simulink library "MotionBaseAdaptersLib"  (R2019b)
settings: Solver=VariableStepAuto  StartTime=0.0  StopTime=10.0  RelTol=1e-3
undefined symbols (not defined in the file): AngularAcceleration, AngularVelocity, ApplyMotion, DiscIntNeverNeededParam, GravitationalAcceleration, LinearAcceleration, LinearVelocity, ManualOrientation, ManualPosition, OrientationDCM, SampleTime, TrackEffectType
libraries: simulink x34, FiltersLib x34, OverridesLib x10, SignalGeneratorsLib x7, LatchesLib x6, TimersLib x5, CoordinateMathOperationsLib x2, MathOperationsLib x2, $bdroot x1
(part 1 of 2)
settings Model: ModifiedComment=azadegaw -- Fri Jun 17 14:06:01 2022 -- Version 1.36  Creator=dward  LastModifiedBy=azadegaw
settings Model: ModifiedHistory=|
  | azadegaw -- Fri Jun 17 14:06:01 2022 -- Version 1.36
  | 
  | azadegaw -- Tue Jun 07 14:53:46 2022 -- Version 1.35
  | added vertical Jolt down.
  | 
  | azadegaw -- Mon Jun 06 18:29:13 2022 -- Version 1.34
  | added absolute to test increase for jolt.
  | multiplied output by input to retain sign,
  | as some jolts are plus and some are minus
  | 
  | staudes -- Thu Apr 21 11:16:42 2022 -- Version 1.33
  | 
  | staudes -- Wed Apr 13 16:31:53 2022 -- Version 1.
  | 
  | staudes -- Thu Apr 07 10:46:09 2022 -- Version 1.31
  | 
  | staudes -- Wed Apr 06 11:32:24 2022 -- Version 1.30
  | Removed Steering Wheel Library
  | 
  | cdyer -- Wed Feb 27 14:51:59 2019 -- Version 1.29
  | - Some modifications to the standard road feel to make it a bit more noticeable
  | - Added logic to lower (and subsequently rampe up) the satuations on accelerations/velocities during collisions
  | - Now set Apply Motion to 0 when Model Data is invalid (mostly handles the extra situation where truksim has stopped the run)
  | 
  | 
  | cdyer -- Wed Feb 20 11:35:48 2019 -- Version 1.28
  | - fixing speed dependent ramp in of motion base effects for raod feel
  | - adding a placeholder for collision gain of motion base outputs
  | 
  | cdyer -- Thu Feb 14 18:34:25 2019 -- Version 1.27
  | -fixed mixup of standard and degraded road feel
  | 
  | cdyer -- Thu Feb 14 12:50:13 2019 -- Version 1.26
  | - Now using the degraded road effect signal to enable the degraded road feel
  | - enabling standard feel by default
  | - road effect may be disabled by setting the profile type to -1.
  | 
  | cdyer -- Wed Jan 16 10:51:13 2019 -- Version 1.25
  | - Adding more complex roughness generation profiles, only enabled by debug properties at this stage
  | 
  | cdyer -- Fri Apr 06 16:05:50 2018 -- Version 1.24
  | -updating default paramaters of steeringwheel adapter for more manageable fualt levels
  | 
  | cdyer -- Thu Feb 15 13:59:35 2018 -- Version 1.23
  | - Adding power steering failure to the effects bus
  | 
  | cdyer -- Mon Jan 22 16:33:43 2018 -- Version 1.22
  | - Upgrading to 2017b
settings DataIOCC: ReturnWorkspaceOutputs=off
settings DebuggingCC: ArithmeticOperatorsInVariantConditions=warning
settings SFSimCC: SimUseLocalCustomCode=off  CustomCodeUndefinedFunction=UseInterfaceOnly
settings RTWCC: RTWUseLocalCustomCode=off
settings CodeAppCC: StateflowObjectComments=on

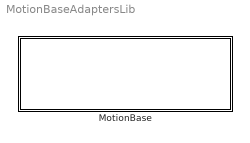
== system MotionBaseAdaptersLib ==
  MotionBase : Subsystem

== system MotionBaseAdaptersLib/MotionBase ==
  MotionBaseAdapter : Subsystem  mask(Motion Base Adapter){}
      mask help: Takes model dynamics data, applies safety limits and outputs motion base control information
  MotionBaseAdaptorInterface : Subsystem

== system MotionBaseAdaptersLib/MotionBase/MotionBaseAdapter ==
  MotionBaseInput : Inport
  Bus to Vector : BusToVector
  MotionBaseProcessing : Subsystem
  SafeMotionBaseOut : Subsystem
  Switch1 : Switch  Criteria=u2 > Threshold
  MotionBaseOutputs : Outport  VectorParamsAs1DForOutWhenUnconnected=off
  StopConditionData : Outport  Port=2  VectorParamsAs1DForOutWhenUnconnected=off
  wires:
  MotionBaseInput/1 -> MotionBaseProcessing/1(MotionBaseInput)
  SafeMotionBaseOut/1(MotionBaseOutputs) -> Switch1/3
  MotionBaseProcessing/1(MotionBaseOutputs) -> Switch1/1
  MotionBaseProcessing/2(AllowMotion) -> Switch1/2
  Switch1/1 -> MotionBaseOutputs/1
  MotionBaseProcessing/3(StopConditionData) -> Bus to Vector/1
  Bus to Vector/1 -> StopConditionData/1

== system MotionBaseAdaptersLib/MotionBase/MotionBaseAdaptorInterface ==
  MotionBaseInput : Inport
  MotionBasePerVehicle : Subsystem
  StopConditionLogging : Subsystem
  MotionBaseOutputs : Outport  VectorParamsAs1DForOutWhenUnconnected=off
  wires:
  MotionBaseInput/1 -> MotionBasePerVehicle/1(MotionBaseInput)
  MotionBasePerVehicle/1(MotionBaseOutputs) -> MotionBaseOutputs/1
  MotionBasePerVehicle/2(StopConditionData) -> StopConditionLogging/1(StopConditionData)

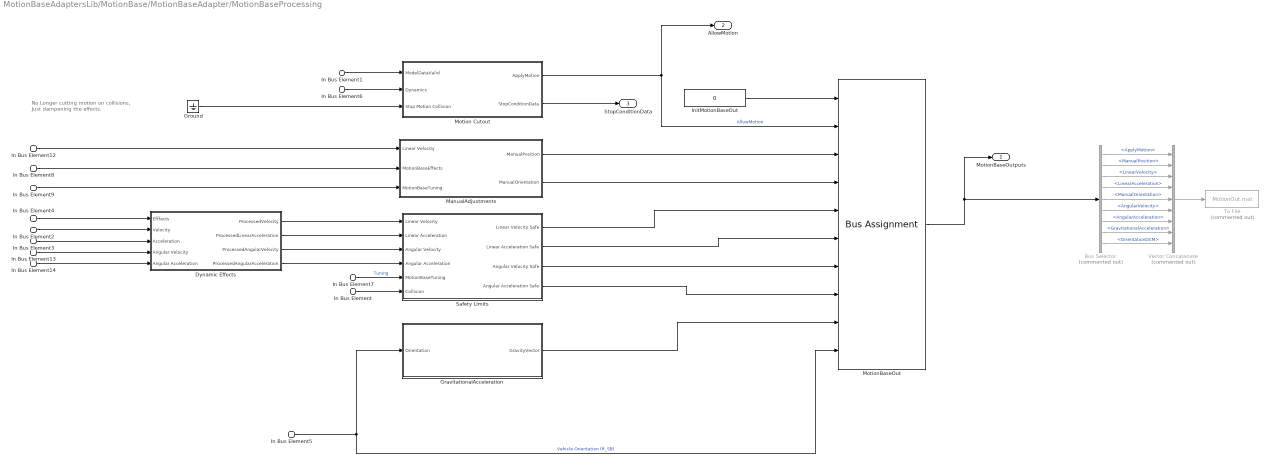
== system MotionBaseAdaptersLib/MotionBase/MotionBaseAdapter/MotionBaseProcessing ==
  note: No Longer cutting motion on collisions,
      | Just dampening the effects.
  In Bus Element : Inport  PortName=MotionBaseInput  Element=Environment.Contact
  In Bus Element6 : Inport  PortName=MotionBaseInput  Element=Dynamics
  In Bus Element12 : Inport  PortName=MotionBaseInput  Element=Dynamics.Velocity
  In Bus Element2 : Inport  PortName=MotionBaseInput  Element=Dynamics.Velocity
  In Bus Element3 : Inport  PortName=MotionBaseInput  Element=Dynamics.Acceleration
  In Bus Element13 : Inport  PortName=MotionBaseInput  Element=Dynamics.AngularVelocity
  In Bus Element14 : Inport  PortName=MotionBaseInput  Element=Dynamics.AngularAcceleration
  In Bus Element5 : Inport  PortName=MotionBaseInput  Element=Dynamics.Transform.OrientationDCM
  In Bus Element4 : Inport  PortName=MotionBaseInput  Element=Effects
  In Bus Element8 : Inport  PortName=MotionBaseInput  Element=Effects.ExternalEffects
  In Bus Element9 : Inport  PortName=MotionBaseInput  Element=Tuning
  In Bus Element7 : Inport  PortName=MotionBaseInput  Element=Tuning
  In Bus Element1 : Inport  PortName=MotionBaseInput  Element=MotionBaseSafetyCutout
  Bus Selector : BusSelector  Commented=on  OutputSignals=ApplyMotion,ManualPosition,LinearVelocity,LinearAcceleration,ManualOrientation,AngularVelocity,AngularAcceleration,GravitationalAcceleration,OrientationDCM
  Dynamic Effects : Subsystem
  GravitationalAcceleration : Subsystem
  Ground : Ground
  InitMotionBaseOut : Constant  Value=0  OutDataTypeStr=Bus: BD_SimIntegration_Out_Vehicle_MotionBaseController
  ManualAdjustments : Subsystem
  Motion Cutout : Subsystem
  MotionBaseOut : BusAssignment  AssignedSignals=ApplyMotion,ManualPosition,ManualOrientation,LinearVelocity,LinearAcceleration,AngularVelocity,AngularAcceleration,GravitationalAcceleration,OrientationDCM
  Safety Limits : Subsystem
  To File : ToFile  Commented=on  Filename=MotionOut.mat  MatrixName=MotionOut
  Vector Concatenate : Concatenate  Commented=on  NumInputs=9
  MotionBaseOutputs : Outport  VectorParamsAs1DForOutWhenUnconnected=off
  AllowMotion : Outport  Port=2  VectorParamsAs1DForOutWhenUnconnected=off
  StopConditionData : Outport  Port=3  VectorParamsAs1DForOutWhenUnconnected=off
  wires:
  In Bus Element1/1 -> Motion Cutout/1(ModelDataValid)
  In Bus Element4/1 -> Dynamic Effects/1(Efffects)
  In Bus Element12/1 -> ManualAdjustments/1(Linear Velocity)
  Dynamic Effects/4(ProcessedAngularAcceleration) -> Safety Limits/4(Angular Acceleration)
  Dynamic Effects/3(ProcessedAngularVelocity) -> Safety Limits/3(Angular Velocity)
  In Bus Element7/1 -> Safety Limits/5(MotionBaseTuning)  "Tuning"
  Dynamic Effects/1(ProcessedVelocity) -> Safety Limits/1(Linear Velocity)
  In Bus Element/1 -> Safety Limits/6(Collision)
  In Bus Element14/1 -> Dynamic Effects/5(Angular Acceleration)
  In Bus Element13/1 -> Dynamic Effects/4(Angular Velocity)
  Dynamic Effects/2(ProcessedLinearAcceleration) -> Safety Limits/2(Linear Acceleration)
  Ground/1 -> Motion Cutout/3(Stop Motion Collision)
  In Bus Element8/1 -> ManualAdjustments/2(MotionBaseEffects)
  In Bus Element9/1 -> ManualAdjustments/3(MotionBaseTuning)
  InitMotionBaseOut/1 -> MotionBaseOut/1
  Motion Cutout/1(ApplyMotion) -> AllowMotion/1, MotionBaseOut/2  "AllowMotion"
  In Bus Element3/1 -> Dynamic Effects/3(Acceleration)
  MotionBaseOut/1 -> Bus Selector/1, MotionBaseOutputs/1
  In Bus Element5/1 -> GravitationalAcceleration/1(Orientation), MotionBaseOut/10  "Vehicle Orientation (R_SB)"
  In Bus Element2/1 -> Dynamic Effects/2(Velocity)
  Safety Limits/1(Linear Velocity Safe) -> MotionBaseOut/5
  Safety Limits/2(Linear Acceleration Safe) -> MotionBaseOut/6
  Safety Limits/3(Angular Velocity Safe) -> MotionBaseOut/7
  Safety Limits/4(Angular Acceleration Safe) -> MotionBaseOut/8
  Bus Selector/5 -> Vector Concatenate/5  "<ManualOrientation>"
  Bus Selector/2 -> Vector Concatenate/2  "<ManualPosition>"
  Bus Selector/4 -> Vector Concatenate/4  "<LinearAcceleration>"
  Bus Selector/6 -> Vector Concatenate/6  "<AngularVelocity>"
  Bus Selector/7 -> Vector Concatenate/7  "<AngularAcceleration>"
  Bus Selector/9 -> Vector Concatenate/9  "<OrientationDCM>"
  Vector Concatenate/1 -> To File/1
  Bus Selector/3 -> Vector Concatenate/3  "<LinearVelocity>"
  Bus Selector/1 -> Vector Concatenate/1  "<ApplyMotion>"
  Bus Selector/8 -> Vector Concatenate/8  "<GravitationalAcceleration>"
  In Bus Element6/1 -> Motion Cutout/2(Dynamics)
  Motion Cutout/2(StopConditionData) -> StopConditionData/1
  GravitationalAcceleration/1(GravityVector) -> MotionBaseOut/9
  ManualAdjustments/1(ManualPosition) -> MotionBaseOut/3
  ManualAdjustments/2(ManualOrientation) -> MotionBaseOut/4

== system MotionBaseAdaptersLib/MotionBase/MotionBaseAdapter/SafeMotionBaseOut ==
  InitMotionBaseOut1 : Constant  Value=0  OutDataTypeStr=Bus: BD_SimIntegration_Out_Vehicle_MotionBaseController
  SafeGravitationalAcceleration : Constant  Value=[0 0 -9.81]
  SafeMotionBaseOut : BusAssignment  AssignedSignals=GravitationalAcceleration,OrientationDCM
  SafeRotationMatrix : Constant  Value=eye(3)
  MotionBaseOutputs : Outport  VectorParamsAs1DForOutWhenUnconnected=off
  wires:
  SafeRotationMatrix/1 -> SafeMotionBaseOut/3
  SafeMotionBaseOut/1 -> MotionBaseOutputs/1  "SafeMotionBaseOut"
  InitMotionBaseOut1/1 -> SafeMotionBaseOut/1
  SafeGravitationalAcceleration/1 -> SafeMotionBaseOut/2

== system MotionBaseAdaptersLib/MotionBase/MotionBaseAdaptorInterface/MotionBasePerVehicle ==
  MotionBaseInput : Inport  Partition=on  PartitionDimension=1  PartitionWidth=1  PartitionOffset=0
  For Each : ForEach  DisableCoverage=on
  MotionBaseAdapter : $bdroot/MotionBase/MotionBaseAdapter
  MotionBaseOutputs : Outport  ConcatenationDimension=1  VectorParamsAs1DForOutWhenUnconnected=off
  StopConditionData : Outport  Port=2  ConcatenationDimension=1  VectorParamsAs1DForOutWhenUnconnected=off
  wires:
  MotionBaseInput/1 -> MotionBaseAdapter/1
  MotionBaseAdapter/2 -> StopConditionData/1
  MotionBaseAdapter/1 -> MotionBaseOutputs/1

== system MotionBaseAdaptersLib/MotionBase/MotionBaseAdaptorInterface/StopConditionLogging ==
  StopConditionData : Inport
  Data Type Conversion : DataTypeConversion
  Demux : Demux  Outputs=5
  Log On Stop Motion : Subsystem  TreatAsAtomicUnit=on
  Vector Concatenate : Concatenate  NumInputs=4
  wires:
  Demux/5 -> Vector Concatenate/4
  Demux/1 -> Log On Stop Motion/Enable
  Demux/4 -> Vector Concatenate/3
  Data Type Conversion/1 -> Log On Stop Motion/1(In1)
  Vector Concatenate/1 -> Data Type Conversion/1
  Demux/2 -> Vector Concatenate/1
  Demux/3 -> Vector Concatenate/2
  StopConditionData/1 -> Demux/1

== system MotionBaseAdaptersLib/MotionBase/MotionBaseAdapter/MotionBaseProcessing/Dynamic Effects ==
  Efffects : Inport
  Velocity : Inport  Port=2
  Acceleration : Inport  Port=3
  Angular Velocity : Inport  Port=4
  Angular Acceleration : Inport  Port=5
  Acceleration Jolts : Subsystem
  ProcessedVelocity : Outport
  ProcessedLinearAcceleration : Outport  Port=2
  ProcessedAngularVelocity : Outport  Port=3
  ProcessedAngularAcceleration : Outport  Port=4
  wires:
  Angular Acceleration/1 -> ProcessedAngularAcceleration/1
  Angular Velocity/1 -> ProcessedAngularVelocity/1
  Velocity/1 -> ProcessedVelocity/1
  Efffects/1 -> Acceleration Jolts/1(Effects)
  Acceleration Jolts/1(AccelerationOut) -> ProcessedLinearAcceleration/1
  Acceleration/1 -> Acceleration Jolts/2(AccelerationIn)

== system MotionBaseAdaptersLib/MotionBase/MotionBaseAdapter/MotionBaseProcessing/GravitationalAcceleration ==
  Orientation : Inport
  DCM Invert : CoordinateMathOperationsLib/DCM Invert
      settings: SourceProductName=Coordinate Systems
  DCM Multiply : CoordinateMathOperationsLib/DCM Multiply
      settings: SourceProductName=Coordinate Systems
  GravitationalAcceleration : Constant  Value=[0 0 -9.81]
  GravityVector : Outport  VectorParamsAs1DForOutWhenUnconnected=off
  wires:
  GravitationalAcceleration/1 -> DCM Multiply/2  "Accleration do to Gravity (V_S)"
  DCM Invert/1 -> DCM Multiply/1  "Vehicle Orientation (R_BS"
  DCM Multiply/1 -> GravityVector/1
  Orientation/1 -> DCM Invert/1

== system MotionBaseAdaptersLib/MotionBase/MotionBaseAdapter/MotionBaseProcessing/ManualAdjustments ==
  Linear Velocity : Inport
  MotionBaseEffects : Inport  Port=2
  MotionBaseTuning : Inport  Port=3
  ManualOrientationAdjustment : Constant  Value=[0 0 0]
  ManualPositionAdjustment : Subsystem
  ManualPositionAdjustment1 : Subsystem  Commented=on
  ManualPosition : Outport  VectorParamsAs1DForOutWhenUnconnected=off
  ManualOrientation : Outport  Port=2  VectorParamsAs1DForOutWhenUnconnected=off
  wires:
  MotionBaseEffects/1 -> ManualPositionAdjustment/2(MotionBaseEffects)
  Linear Velocity/1 -> ManualPositionAdjustment/1(Linear Velocity)
  MotionBaseTuning/1 -> ManualPositionAdjustment/3(MotionBaseTuning)
  ManualOrientationAdjustment/1 -> ManualOrientation/1  "ManualOrientation"
  ManualPositionAdjustment/1(ManualPosition) -> ManualPosition/1  "ManualPosition"

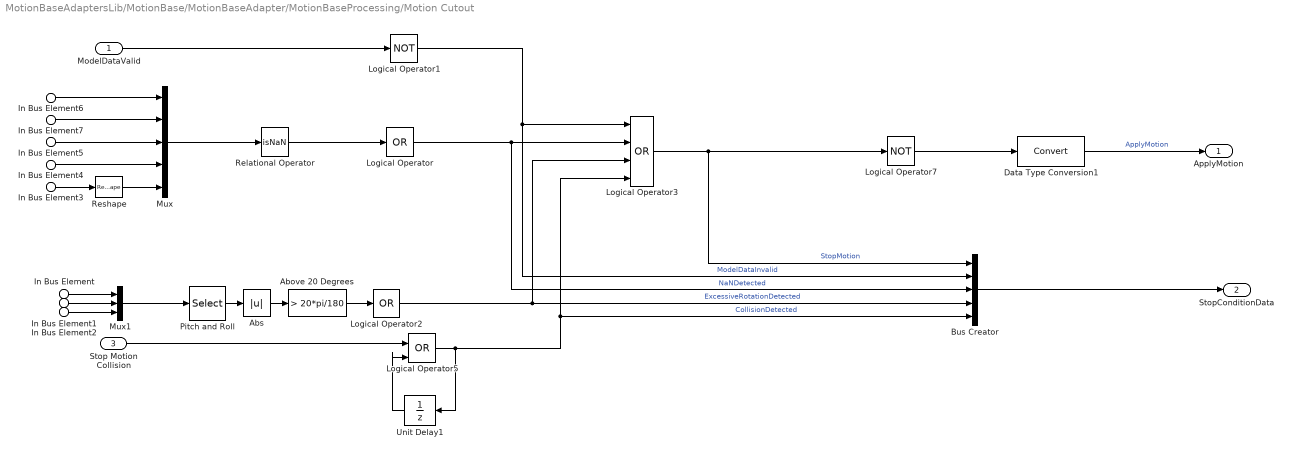
== system MotionBaseAdaptersLib/MotionBase/MotionBaseAdapter/MotionBaseProcessing/Motion Cutout ==
  ModelDataValid : Inport
  In Bus Element : Inport  Port=2  PortName=Dynamics  Element=Transform.H
  In Bus Element1 : Inport  Port=2  PortName=Dynamics  Element=Transform.P
  In Bus Element2 : Inport  Port=2  PortName=Dynamics  Element=Transform.R
  In Bus Element3 : Inport  Port=2  PortName=Dynamics  Element=Transform.OrientationDCM
  In Bus Element4 : Inport  Port=2  PortName=Dynamics  Element=AngularAcceleration
  In Bus Element5 : Inport  Port=2  PortName=Dynamics  Element=AngularVelocity
  In Bus Element6 : Inport  Port=2  PortName=Dynamics  Element=Velocity
  In Bus Element7 : Inport  Port=2  PortName=Dynamics  Element=Acceleration
  Stop Motion Collision : Inport  Port=3
  Above 20 Degrees : simulink/Logic and Bit Operations/Compare To Constant  relop=>  const=20*pi/180  OutDataTypeStr=boolean
  Abs : Abs
  Bus Creator : BusCreator  Inputs=5
  Data Type Conversion1 : DataTypeConversion
  Logical Operator : Logic  Operator=OR  Inputs=1  IconShape=distinctive  AllPortsSameDT=off  OutDataTypeStr=boolean
  Logical Operator1 : Logic  Operator=NOT  IconShape=distinctive  AllPortsSameDT=off  OutDataTypeStr=boolean
  Logical Operator2 : Logic  Operator=OR  Inputs=1  IconShape=distinctive  AllPortsSameDT=off  OutDataTypeStr=boolean
  Logical Operator3 : Logic  Operator=OR  Inputs=4  IconShape=distinctive  AllPortsSameDT=off  OutDataTypeStr=boolean
  Logical Operator5 : Logic  Operator=OR  IconShape=distinctive  AllPortsSameDT=off  OutDataTypeStr=boolean
  Logical Operator7 : Logic  Operator=NOT  IconShape=distinctive  AllPortsSameDT=off  OutDataTypeStr=boolean
  Mux : Mux  Inputs=[3 3 3 3 9]
  Mux1 : Mux  Inputs=3
  Pitch and Roll : Selector  InputPortWidth=3  IndexOptions=Index vector (dialog)  Indices=[2 3]  OutputSizes=1
  Relational Operator : RelationalOperator  Operator=isNaN  OutDataTypeStr=boolean  RndMeth=Nearest
  Reshape : Reshape
  Unit Delay1 : UnitDelay  SampleTime=-1  HasFrameUpgradeWarning=on
  ApplyMotion : Outport  VectorParamsAs1DForOutWhenUnconnected=off
  StopConditionData : Outport  Port=2  VectorParamsAs1DForOutWhenUnconnected=off
  wires:
  Logical Operator1/1 -> Logical Operator3/1, Bus Creator/2  "ModelDataInvalid"
  ModelDataValid/1 -> Logical Operator1/1
  Stop Motion Collision/1 -> Logical Operator5/1
  Logical Operator3/1 -> Bus Creator/1, Logical Operator7/1  "StopMotion"
  Mux/1 -> Relational Operator/1
  Relational Operator/1 -> Logical Operator/1
  Logical Operator/1 -> Bus Creator/3, Logical Operator3/2  "NaNDetected"
  In Bus Element6/1 -> Mux/1
  In Bus Element5/1 -> Mux/3
  In Bus Element3/1 -> Reshape/1
  In Bus Element4/1 -> Mux/4
  In Bus Element7/1 -> Mux/2
  Abs/1 -> Above 20 Degrees/1
  Above 20 Degrees/1 -> Logical Operator2/1
  Logical Operator2/1 -> Bus Creator/4, Logical Operator3/3  "ExcessiveRotationDetected"
  Pitch and Roll/1 -> Abs/1
  Logical Operator5/1 -> Unit Delay1/1, Bus Creator/5, Logical Operator3/4  "CollisionDetected"
  Unit Delay1/1 -> Logical Operator5/2
  Logical Operator7/1 -> Data Type Conversion1/1
  Data Type Conversion1/1 -> ApplyMotion/1  "ApplyMotion"
  In Bus Element2/1 -> Mux1/3
  In Bus Element1/1 -> Mux1/2
  In Bus Element/1 -> Mux1/1
  Mux1/1 -> Pitch and Roll/1
  Reshape/1 -> Mux/5
  Bus Creator/1 -> StopConditionData/1

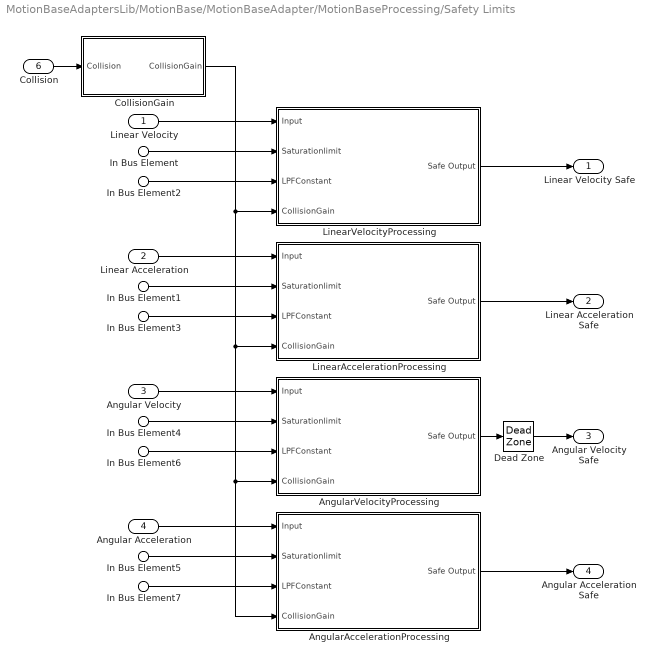
== system MotionBaseAdaptersLib/MotionBase/MotionBaseAdapter/MotionBaseProcessing/Safety Limits ==
  Linear Velocity : Inport
  Linear Acceleration : Inport  Port=2
  Angular Velocity : Inport  Port=3
  Angular Acceleration : Inport  Port=4
  In Bus Element : Inport  Port=5  PortName=MotionBaseTuning  Element=LinearVelocitySaturation
  In Bus Element1 : Inport  Port=5  PortName=MotionBaseTuning  Element=LinearAccelerationSaturation
  In Bus Element2 : Inport  Port=5  PortName=MotionBaseTuning  Element=LinearVelocityLPFConstant
  In Bus Element3 : Inport  Port=5  PortName=MotionBaseTuning  Element=LinearAccelerationLPFConstant
  In Bus Element4 : Inport  Port=5  PortName=MotionBaseTuning  Element=AngularVelocitySaturation
  In Bus Element5 : Inport  Port=5  PortName=MotionBaseTuning  Element=AngularAccelerationSaturation
  In Bus Element6 : Inport  Port=5  PortName=MotionBaseTuning  Element=AngularVelocityLPFConstant
  In Bus Element7 : Inport  Port=5  PortName=MotionBaseTuning  Element=AngularAccelerationLPFConstant
  Collision : Inport  Port=6
  AngularAccelerationProcessing : Subsystem
  AngularVelocityProcessing : Subsystem
  CollisionGain : Subsystem
  Dead Zone : DeadZone  LowerValue=-1e-05  UpperValue=1e-05  SaturateOnIntegerOverflow=on
  LinearAccelerationProcessing : Subsystem
  LinearVelocityProcessing : Subsystem
  Linear Velocity Safe : Outport  VectorParamsAs1DForOutWhenUnconnected=off
  Linear Acceleration Safe : Outport  Port=2  VectorParamsAs1DForOutWhenUnconnected=off
  Angular Velocity Safe : Outport  Port=3  VectorParamsAs1DForOutWhenUnconnected=off
  Angular Acceleration Safe : Outport  Port=4  VectorParamsAs1DForOutWhenUnconnected=off
  wires:
  Collision/1 -> CollisionGain/1(Collision)
  CollisionGain/1(CollisionGain) -> LinearAccelerationProcessing/4(CollisionGain), AngularAccelerationProcessing/4(CollisionGain), AngularVelocityProcessing/4(CollisionGain), LinearVelocityProcessing/4(CollisionGain)
  In Bus Element7/1 -> AngularAccelerationProcessing/3(LPFConstant)
  In Bus Element6/1 -> AngularVelocityProcessing/3(LPFConstant)
  In Bus Element5/1 -> AngularAccelerationProcessing/2(Saturationlimit)
  In Bus Element4/1 -> AngularVelocityProcessing/2(Saturationlimit)
  In Bus Element1/1 -> LinearAccelerationProcessing/2(Saturationlimit)
  In Bus Element/1 -> LinearVelocityProcessing/2(Saturationlimit)
  Linear Velocity/1 -> LinearVelocityProcessing/1(Input)
  In Bus Element2/1 -> LinearVelocityProcessing/3(LPFConstant)
  LinearVelocityProcessing/1(Safe Output) -> Linear Velocity Safe/1
  In Bus Element3/1 -> LinearAccelerationProcessing/3(LPFConstant)
  Linear Acceleration/1 -> LinearAccelerationProcessing/1(Input)
  LinearAccelerationProcessing/1(Safe Output) -> Linear Acceleration Safe/1
  Angular Velocity/1 -> AngularVelocityProcessing/1(Input)
  AngularVelocityProcessing/1(Safe Output) -> Dead Zone/1
  Dead Zone/1 -> Angular Velocity Safe/1
  AngularAccelerationProcessing/1(Safe Output) -> Angular Acceleration Safe/1
  Angular Acceleration/1 -> AngularAccelerationProcessing/1(Input)

== system MotionBaseAdaptersLib/MotionBase/MotionBaseAdaptorInterface/StopConditionLogging/Log On Stop Motion ==
  In1 : Inport
  Enable : EnablePort
  To File : ToFile  Filename=MotionStop.mat  MatrixName=MotionStop
  wires:
  In1/1 -> To File/1

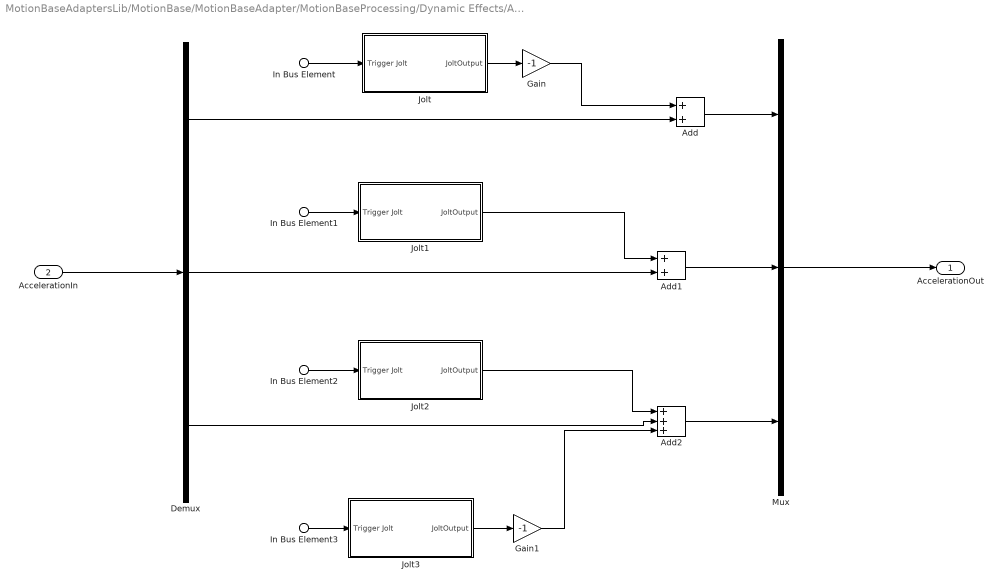
== system MotionBaseAdaptersLib/MotionBase/MotionBaseAdapter/MotionBaseProcessing/Dynamic Effects/Acceleration Jolts ==
  In Bus Element : Inport  PortName=Effects  Element=LongitudinalJolt
  In Bus Element1 : Inport  PortName=Effects  Element=LateralJolt
  In Bus Element2 : Inport  PortName=Effects  Element=VerticalJolt
  In Bus Element3 : Inport  PortName=Effects  Element=VerticalJoltDown
  AccelerationIn : Inport  Port=2
  Add : Sum
  Add1 : Sum
  Add2 : Sum  Inputs=+++
  Demux : Demux  Outputs=3
  Gain : Gain  Gain=-1
  Gain1 : Gain  Gain=-1
  Jolt : Subsystem  mask{Duration=0.5, JoltProfile=[0, 1.5, 2, 1.8, 1.5, 0], JoltBreakPoints=[0, 0.1, 0.2, 0.3, 0.4, 0.5]}
      mask prompts: Duration "Duration of Jolt"; JoltProfile "Jolt Profile Curve"; JoltBreakPoints "Jolt Breakpoints"
      mask help:
      | Creates a disturbance with a specified profile upon a rising edge of the input.
      |
      | Duration must be equal to the end time specified in the Jolt Breakpoints in order for the signal to work correctly
  Jolt1 : Subsystem  mask{Duration=0.5, JoltProfile=[0, 1.5, 2, 1.8, 1.5, 0], JoltBreakPoints=[0, 0.1, 0.2, 0.3, 0.4, 0.5]}
      mask prompts: Duration "Duration of Jolt"; JoltProfile "Jolt Profile Curve"; JoltBreakPoints "Jolt Breakpoints"
      mask help:
      | Creates a disturbance with a specified profile upon a rising edge of the input.
      |
      | Duration must be equal to the end time specified in the Jolt Breakpoints in order for the signal to work correctly
  Jolt2 : Subsystem  mask{Duration=0.5, JoltProfile=[0, 1.5, 2, 1.8, 1.5, 0], JoltBreakPoints=[0, 0.1, 0.2, 0.3, 0.4, 0.5]}
      mask prompts: Duration "Duration of Jolt"; JoltProfile "Jolt Profile Curve"; JoltBreakPoints "Jolt Breakpoints"
      mask help:
      | Creates a disturbance with a specified profile upon a rising edge of the input.
      |
      | Duration must be equal to the end time specified in the Jolt Breakpoints in order for the signal to work correctly
  Jolt3 : Subsystem  mask{Duration=0.5, JoltProfile=[0, 1.5, 2, 1.8, 1.5, 0], JoltBreakPoints=[0, 0.1, 0.2, 0.3, 0.4, 0.5]}
      mask prompts: Duration "Duration of Jolt"; JoltProfile "Jolt Profile Curve"; JoltBreakPoints "Jolt Breakpoints"
      mask help:
      | Creates a disturbance with a specified profile upon a rising edge of the input.
      |
      | Duration must be equal to the end time specified in the Jolt Breakpoints in order for the signal to work correctly
  Mux : Mux  Inputs=3
  AccelerationOut : Outport
  wires:
  Gain1/1 -> Add2/3
  Jolt3/1(JoltOutput) -> Gain1/1
  In Bus Element3/1 -> Jolt3/1(Trigger Jolt)
  Jolt2/1(JoltOutput) -> Add2/1
  Jolt1/1(JoltOutput) -> Add1/1
  Gain/1 -> Add/1
  Jolt/1(JoltOutput) -> Gain/1
  In Bus Element2/1 -> Jolt2/1(Trigger Jolt)
  In Bus Element1/1 -> Jolt1/1(Trigger Jolt)
  In Bus Element/1 -> Jolt/1(Trigger Jolt)
  Mux/1 -> AccelerationOut/1
  AccelerationIn/1 -> Demux/1
  Add2/1 -> Mux/3
  Add/1 -> Mux/1
  Add1/1 -> Mux/2
  Demux/1 -> Add/2
  Demux/2 -> Add1/2
  Demux/3 -> Add2/2

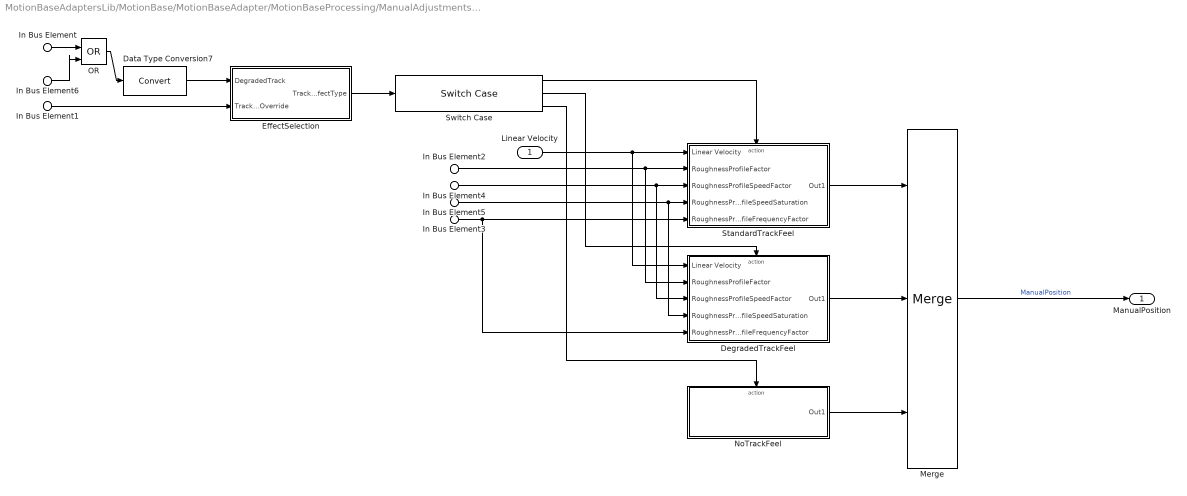
== system MotionBaseAdaptersLib/MotionBase/MotionBaseAdapter/MotionBaseProcessing/ManualAdjustments/ManualPositionAdjustment ==
  Linear Velocity : Inport
  In Bus Element6 : Inport  Port=2  PortName=MotionBaseEffects  Element=DegradedTrack
  In Bus Element : Inport  Port=2  PortName=MotionBaseEffects  Element=OnRoughTrack
  In Bus Element2 : Inport  Port=3  PortName=MotionBaseTuning  Element=RoughnessProfileFactor
  In Bus Element1 : Inport  Port=3  PortName=MotionBaseTuning  Element=RoughnessProfileType
  In Bus Element3 : Inport  Port=3  PortName=MotionBaseTuning  Element=RoughnessProfileFrequencyFactor
  In Bus Element4 : Inport  Port=3  PortName=MotionBaseTuning  Element=RoughnessProfileSpeedFactor
  In Bus Element5 : Inport  Port=3  PortName=MotionBaseTuning  Element=RoughnessProfileSpeedSaturation
  Data Type Conversion7 : DataTypeConversion
  DegradedTrackFeel : Subsystem  TreatAsAtomicUnit=on
  EffectSelection : Subsystem
  Merge : Merge  Inputs=3
  NoTrackFeel : Subsystem  TreatAsAtomicUnit=on
  OR : Logic  Operator=OR  IconShape=distinctive  AllPortsSameDT=off  OutDataTypeStr=boolean
  StandardTrackFeel : Subsystem  TreatAsAtomicUnit=on
  Switch Case : SwitchCase  CaseConditions={TrackEffectType.StandardTrack, TrackEffectType.DegradedTrack, TrackEffectType.NoTrackEffect}  ShowDefaultCase=off
  ManualPosition : Outport  VectorParamsAs1DForOutWhenUnconnected=off
  wires:
  Data Type Conversion7/1 -> EffectSelection/1(DegradedTrack)
  OR/1 -> Data Type Conversion7/1
  In Bus Element/1 -> OR/1
  EffectSelection/1(TrackEffectType) -> Switch Case/1
  In Bus Element6/1 -> OR/2
  In Bus Element1/1 -> EffectSelection/2(TrackEffectOverride)
  Switch Case/2 -> DegradedTrackFeel/Action
  In Bus Element3/1 -> StandardTrackFeel/5(RoughnessProfileFrequencyFactor), DegradedTrackFeel/5(RoughnessProfileFrequencyFactor)
  Linear Velocity/1 -> StandardTrackFeel/1(Linear Velocity), DegradedTrackFeel/1(Linear Velocity)
  DegradedTrackFeel/1(Out1) -> Merge/2
  In Bus Element5/1 -> StandardTrackFeel/4(RoughnessProfileSpeedSaturation), DegradedTrackFeel/4(RoughnessProfileSpeedSaturation)
  In Bus Element4/1 -> StandardTrackFeel/3(RoughnessProfileSpeedFactor), DegradedTrackFeel/3(RoughnessProfileSpeedFactor)
  StandardTrackFeel/1(Out1) -> Merge/1
  In Bus Element2/1 -> StandardTrackFeel/2(RoughnessProfileFactor), DegradedTrackFeel/2(RoughnessProfileFactor)
  NoTrackFeel/1(Out1) -> Merge/3
  Switch Case/3 -> NoTrackFeel/Action
  Switch Case/1 -> StandardTrackFeel/Action
  Merge/1 -> ManualPosition/1  "ManualPosition"

== system MotionBaseAdaptersLib/MotionBase/MotionBaseAdapter/MotionBaseProcessing/ManualAdjustments/ManualPositionAdjustment1 ==
  Linear Velocity : Inport
  In Bus Element2 : Inport  Port=2  PortName=MotionBaseTuning  Element=RoughnessProfileFactor
  In Bus Element1 : Inport  Port=2  PortName=MotionBaseTuning  Element=RoughnessProfileType
  In Bus Element3 : Inport  Port=2  PortName=MotionBaseTuning  Element=RoughnessProfileFrequencyFactor
  In Bus Element4 : Inport  Port=2  PortName=MotionBaseTuning  Element=RoughnessProfileSpeedFactor
  In Bus Element5 : Inport  Port=2  PortName=MotionBaseTuning  Element=RoughnessProfileSpeedSaturation
  If : If  IfExpression=u1 == 1  ElseIfExpressions=u1 == 2,u1 == 3,u1 == 4
  If Action Subsystem : Subsystem  TreatAsAtomicUnit=on
  If Action Subsystem1 : Subsystem  TreatAsAtomicUnit=on
  If Action Subsystem2 : Subsystem  TreatAsAtomicUnit=on
  If Action Subsystem3 : Subsystem  Commented=on  TreatAsAtomicUnit=on
  If Action Subsystem4 : Subsystem  Commented=on  TreatAsAtomicUnit=on
  If Action Subsystem5 : Subsystem  TreatAsAtomicUnit=on
  If Action Subsystem6 : Subsystem  TreatAsAtomicUnit=on
  Merge : Merge  Inputs=5
  ManualPosition : Outport  VectorParamsAs1DForOutWhenUnconnected=off
  wires:
  Merge/1 -> ManualPosition/1  "ManualPosition"
  In Bus Element1/1 -> If/1
  If/1 -> If Action Subsystem/Action
  If/2 -> If Action Subsystem1/Action
  If/5 -> If Action Subsystem2/Action
  If Action Subsystem/1(Out1) -> Merge/1
  If Action Subsystem1/1(Out1) -> Merge/2
  If Action Subsystem2/1(Out1) -> Merge/5
  In Bus Element2/1 -> If Action Subsystem6/2(RoughnessProfileFactor), If Action Subsystem5/2(RoughnessProfileFactor), If Action Subsystem1/2(RoughnessProfileFactor), If Action Subsystem/2(RoughnessProfileFactor)
  If/3 -> If Action Subsystem5/Action
  If Action Subsystem5/1(Out1) -> Merge/3
  In Bus Element4/1 -> If Action Subsystem6/3(RoughnessProfileSpeedFactor), If Action Subsystem5/3(RoughnessProfileSpeedFactor), If Action Subsystem1/3(RoughnessProfileSpeedFactor), If Action Subsystem/3(RoughnessProfileSpeedFactor)
  In Bus Element5/1 -> If Action Subsystem6/4(RoughnessProfileSpeedSaturation), If Action Subsystem5/4(RoughnessProfileSpeedSaturation), If Action Subsystem1/4(RoughnessProfileSpeedSaturation), If Action Subsystem/4(RoughnessProfileSpeedSaturation)
  If/4 -> If Action Subsystem6/Action
  If Action Subsystem6/1(Out1) -> Merge/4
  Linear Velocity/1 -> If Action Subsystem5/1(Linear Velocity), If Action Subsystem6/1(Linear Velocity), If Action Subsystem1/1(Linear Velocity), If Action Subsystem/1(Linear Velocity)
  In Bus Element3/1 -> If Action Subsystem/5(RoughnessProfileFrequencyFactor), If Action Subsystem1/5(RoughnessProfileFrequencyFactor), If Action Subsystem5/5(RoughnessProfileFrequencyFactor), If Action Subsystem6/5(RoughnessProfileFrequencyFactor)

== system MotionBaseAdaptersLib/MotionBase/MotionBaseAdapter/MotionBaseProcessing/Safety Limits/AngularAccelerationProcessing ==
  Input : Inport
  Saturationlimit : Inport  Port=2
  LPFConstant : Inport  Port=3
  CollisionGain : Inport  Port=4
  1-D Lookup Table : Lookup_n-D  NumberOfTableDimensions=1  BreakpointsForDimension1=[.1 1]  Table=[.5 1]  ExtrapMethod=Clip  UseLastTableValue=on  InternalRulePriority=Speed  RndMeth=Simplest  InputSameDT=on
  First Order Low Pass Filter : FiltersLib/First Order Low Pass Filter  FilterSpecificationSource=external  FilterSpecificationType=Specify Cutoff Frequency  FilterSpecificationValue=0.01  SampleTime=-1
      settings: SourceProductName=Filters
  Gain : Gain  Gain=-1
  LPFConstantTuning : OverridesLib/Tuning Factor  DefaultValue=4.5  Criteria=u2 > Threshold  Threshold=0
      settings: SourceProductName=Sydac Utilities
  Product : Product
  Saturation Dynamic : simulink/Discontinuities/Saturation Dynamic  OutMin=[]  OutMax=[]  OutDataTypeStr=Inherit: Same as second input  OutDataType=fixdt(1, 16)  OutScaling=2^-10  DoSatur=off
  SaturationTuning : OverridesLib/Tuning Factor  DefaultValue=2  Criteria=u2 > Threshold  Threshold=0
      settings: SourceProductName=Sydac Utilities
  Safe Output : Outport  VectorParamsAs1DForOutWhenUnconnected=off
  wires:
  1-D Lookup Table/1 -> Product/1
  SaturationTuning/1 -> Product/2
  CollisionGain/1 -> 1-D Lookup Table/1
  LPFConstantTuning/1 -> First Order Low Pass Filter/2
  Saturation Dynamic/1 -> Safe Output/1
  First Order Low Pass Filter/1 -> Saturation Dynamic/2
  Saturationlimit/1 -> SaturationTuning/1
  LPFConstant/1 -> LPFConstantTuning/1
  Input/1 -> First Order Low Pass Filter/1
  Product/1 -> Gain/1, Saturation Dynamic/1
  Gain/1 -> Saturation Dynamic/3

== system MotionBaseAdaptersLib/MotionBase/MotionBaseAdapter/MotionBaseProcessing/Safety Limits/AngularVelocityProcessing ==
  Input : Inport
  Saturationlimit : Inport  Port=2
  LPFConstant : Inport  Port=3
  CollisionGain : Inport  Port=4
  1-D Lookup Table : Lookup_n-D  NumberOfTableDimensions=1  BreakpointsForDimension1=[.1 1]  Table=[.4 1]  ExtrapMethod=Clip  UseLastTableValue=on  InternalRulePriority=Speed  RndMeth=Simplest  InputSameDT=on
  First Order Low Pass Filter : FiltersLib/First Order Low Pass Filter  FilterSpecificationSource=external  FilterSpecificationType=Specify Cutoff Frequency  FilterSpecificationValue=0.01  SampleTime=-1
      settings: SourceProductName=Filters
  Gain : Gain  Gain=-1
  LPFConstantTuning : OverridesLib/Tuning Factor  DefaultValue=10  Criteria=u2 > Threshold  Threshold=0
      settings: SourceProductName=Sydac Utilities
  Product : Product
  Saturation Dynamic : simulink/Discontinuities/Saturation Dynamic  OutMin=[]  OutMax=[]  OutDataTypeStr=Inherit: Same as second input  OutDataType=fixdt(1, 16)  OutScaling=2^-10  DoSatur=off
  SaturationTuning : OverridesLib/Tuning Factor  DefaultValue=2  Criteria=u2 > Threshold  Threshold=0
      settings: SourceProductName=Sydac Utilities
  Safe Output : Outport  VectorParamsAs1DForOutWhenUnconnected=off
  wires:
  1-D Lookup Table/1 -> Product/1
  CollisionGain/1 -> 1-D Lookup Table/1
  SaturationTuning/1 -> Product/2
  LPFConstantTuning/1 -> First Order Low Pass Filter/2
  Saturation Dynamic/1 -> Safe Output/1
  First Order Low Pass Filter/1 -> Saturation Dynamic/2
  Saturationlimit/1 -> SaturationTuning/1
  LPFConstant/1 -> LPFConstantTuning/1
  Input/1 -> First Order Low Pass Filter/1
  Product/1 -> Gain/1, Saturation Dynamic/1
  Gain/1 -> Saturation Dynamic/3

== system MotionBaseAdaptersLib/MotionBase/MotionBaseAdapter/MotionBaseProcessing/Safety Limits/CollisionGain ==
  note: May be able to try and dampen the motion base repsonse during an active collision,
      | and slowly ramp back up to full response over time after the collision.
  Collision : Inport
  CollisionGainReset : Constant  Value=0.1
  Discrete-Time Integrator : DiscreteIntegrator  ExternalReset=level  InitialConditionSource=external  InitialCondition=1  SampleTime=-1  LimitOutput=on  UpperSaturationLimit=1  LowerSaturationLimit=0  ICPrevOutput=DiscIntNeverNeededParam  ICPrevScaledInput=DiscIntNeverNeededParam
  IC : InitialCondition
  RampRate : Constant  Value=1/5
  TimerOffDelay NoInit : TimersLib/TimerOffDelay NoInit  UpperSaturationLimit=2  SampleTime=-1
      settings: SourceProductName=Sydac Utilities
  CollisionGain : Outport  VectorParamsAs1DForOutWhenUnconnected=off
  wires:
  TimerOffDelay NoInit/1 -> Discrete-Time Integrator/2
  Discrete-Time Integrator/1 -> CollisionGain/1
  Collision/1 -> TimerOffDelay NoInit/1
  IC/1 -> Discrete-Time Integrator/3
  CollisionGainReset/1 -> IC/1
  RampRate/1 -> Discrete-Time Integrator/1

== system MotionBaseAdaptersLib/MotionBase/MotionBaseAdapter/MotionBaseProcessing/Safety Limits/LinearAccelerationProcessing ==
  Input : Inport
  Saturationlimit : Inport  Port=2
  LPFConstant : Inport  Port=3
  CollisionGain : Inport  Port=4
  First Order Low Pass Filter : FiltersLib/First Order Low Pass Filter  FilterSpecificationSource=external  FilterSpecificationType=Specify Cutoff Frequency  FilterSpecificationValue=0.01  SampleTime=-1
      settings: SourceProductName=Filters
  Gain : Gain  Gain=-1
  LPFConstantTuning : OverridesLib/Tuning Factor  DefaultValue=4.5  Criteria=u2 > Threshold  Threshold=0
      settings: SourceProductName=Sydac Utilities
  Product : Product
  Saturation Dynamic : simulink/Discontinuities/Saturation Dynamic  OutMin=[]  OutMax=[]  OutDataTypeStr=Inherit: Same as second input  OutDataType=fixdt(1, 16)  OutScaling=2^-10  DoSatur=off
  SaturationTuning : OverridesLib/Tuning Factor  DefaultValue=10  Criteria=u2 > Threshold  Threshold=0
      settings: SourceProductName=Sydac Utilities
  Safe Output : Outport  VectorParamsAs1DForOutWhenUnconnected=off
  wires:
  CollisionGain/1 -> Product/1
  SaturationTuning/1 -> Product/2
  Gain/1 -> Saturation Dynamic/3
  Product/1 -> Saturation Dynamic/1, Gain/1
  Input/1 -> First Order Low Pass Filter/1
  LPFConstant/1 -> LPFConstantTuning/1
  Saturationlimit/1 -> SaturationTuning/1
  First Order Low Pass Filter/1 -> Saturation Dynamic/2
  Saturation Dynamic/1 -> Safe Output/1
  LPFConstantTuning/1 -> First Order Low Pass Filter/2

== system MotionBaseAdaptersLib/MotionBase/MotionBaseAdapter/MotionBaseProcessing/Safety Limits/LinearVelocityProcessing ==
  Input : Inport
  Saturationlimit : Inport  Port=2
  LPFConstant : Inport  Port=3
  CollisionGain : Inport  Port=4
  1-D Lookup Table : Lookup_n-D  NumberOfTableDimensions=1  BreakpointsForDimension1=[.1 1]  Table=[.01 1]  ExtrapMethod=Clip  UseLastTableValue=on  InternalRulePriority=Speed  RndMeth=Simplest  InputSameDT=on
  First Order Low Pass Filter : FiltersLib/First Order Low Pass Filter  FilterSpecificationSource=external  FilterSpecificationType=Specify Cutoff Frequency  FilterSpecificationValue=0.01  SampleTime=-1
      settings: SourceProductName=Filters
  Gain : Gain  Gain=-1
  LPFConstantTuning : OverridesLib/Tuning Factor  DefaultValue=10  Criteria=u2 > Threshold  Threshold=0
      settings: SourceProductName=Sydac Utilities
  Product : Product
  Saturation Dynamic : simulink/Discontinuities/Saturation Dynamic  OutMin=[]  OutMax=[]  OutDataTypeStr=Inherit: Same as second input  OutDataType=fixdt(1, 16)  OutScaling=2^-10  DoSatur=off
  SaturationTuning : OverridesLib/Tuning Factor  DefaultValue=50  Criteria=u2 > Threshold  Threshold=0
      settings: SourceProductName=Sydac Utilities
  Safe Output : Outport  VectorParamsAs1DForOutWhenUnconnected=off
  wires:
  1-D Lookup Table/1 -> Product/1
  CollisionGain/1 -> 1-D Lookup Table/1
  SaturationTuning/1 -> Product/2
  LPFConstantTuning/1 -> First Order Low Pass Filter/2
  Saturation Dynamic/1 -> Safe Output/1
  First Order Low Pass Filter/1 -> Saturation Dynamic/2
  Saturationlimit/1 -> SaturationTuning/1
  LPFConstant/1 -> LPFConstantTuning/1
  Input/1 -> First Order Low Pass Filter/1
  Product/1 -> Gain/1, Saturation Dynamic/1
  Gain/1 -> Saturation Dynamic/3

== system MotionBaseAdaptersLib/MotionBase/MotionBaseAdapter/MotionBaseProcessing/Dynamic Effects/Acceleration Jolts/Jolt ==
  Trigger Jolt : Inport
  Data Type Conversion : DataTypeConversion
  Detect Increase : simulink/Logic and Bit Operations/Detect Increase  vinit=0.0  OutDataTypeStr=boolean
  Discrete-Time Integrator : DiscreteIntegrator  ExternalReset=falling  SampleTime=-1  ICPrevOutput=DiscIntNeverNeededParam  ICPrevScaledInput=DiscIntNeverNeededParam
  Jolt Duration : TimersLib/TimerOffDelay NoInit  UpperSaturationLimit=Duration  SampleTime=-1
      settings: SourceProductName=Sydac Utilities
  Jolt Profile : Lookup_n-D  NumberOfTableDimensions=1  BreakpointsForDimension1=JoltBreakPoints  Table=JoltProfile  ExtrapMethod=Clip  InternalRulePriority=Speed  RndMeth=Simplest  InputSameDT=on
  JoltOutput : Outport
  wires:
  Trigger Jolt/1 -> Detect Increase/1
  Data Type Conversion/1 -> Discrete-Time Integrator/1
  Jolt Duration/1 -> Discrete-Time Integrator/2, Data Type Conversion/1
  Jolt Profile/1 -> JoltOutput/1
  Discrete-Time Integrator/1 -> Jolt Profile/1
  Detect Increase/1 -> Jolt Duration/1

== system MotionBaseAdaptersLib/MotionBase/MotionBaseAdapter/MotionBaseProcessing/Dynamic Effects/Acceleration Jolts/Jolt1 ==
  Trigger Jolt : Inport
  Data Type Conversion : DataTypeConversion
  Detect Increase : simulink/Logic and Bit Operations/Detect Increase  vinit=0.0  OutDataTypeStr=boolean
  Discrete-Time Integrator : DiscreteIntegrator  ExternalReset=falling  SampleTime=-1  ICPrevOutput=DiscIntNeverNeededParam  ICPrevScaledInput=DiscIntNeverNeededParam
  Jolt Duration : TimersLib/TimerOffDelay NoInit  UpperSaturationLimit=Duration  SampleTime=-1
      settings: SourceProductName=Sydac Utilities
  Jolt Profile : Lookup_n-D  NumberOfTableDimensions=1  BreakpointsForDimension1=JoltBreakPoints  Table=JoltProfile  ExtrapMethod=Clip  InternalRulePriority=Speed  RndMeth=Simplest  InputSameDT=on
  JoltOutput : Outport
  wires:
  Trigger Jolt/1 -> Detect Increase/1
  Data Type Conversion/1 -> Discrete-Time Integrator/1
  Jolt Duration/1 -> Discrete-Time Integrator/2, Data Type Conversion/1
  Jolt Profile/1 -> JoltOutput/1
  Discrete-Time Integrator/1 -> Jolt Profile/1
  Detect Increase/1 -> Jolt Duration/1

== system MotionBaseAdaptersLib/MotionBase/MotionBaseAdapter/MotionBaseProcessing/Dynamic Effects/Acceleration Jolts/Jolt2 ==
  Trigger Jolt : Inport
  Data Type Conversion : DataTypeConversion
  Detect Increase : simulink/Logic and Bit Operations/Detect Increase  vinit=0.0  OutDataTypeStr=boolean
  Discrete-Time Integrator : DiscreteIntegrator  ExternalReset=falling  SampleTime=-1  ICPrevOutput=DiscIntNeverNeededParam  ICPrevScaledInput=DiscIntNeverNeededParam
  Jolt Duration : TimersLib/TimerOffDelay NoInit  UpperSaturationLimit=Duration  SampleTime=-1
      settings: SourceProductName=Sydac Utilities
  Jolt Profile : Lookup_n-D  NumberOfTableDimensions=1  BreakpointsForDimension1=JoltBreakPoints  Table=JoltProfile  ExtrapMethod=Clip  InternalRulePriority=Speed  RndMeth=Simplest  InputSameDT=on
  JoltOutput : Outport
  wires:
  Trigger Jolt/1 -> Detect Increase/1
  Data Type Conversion/1 -> Discrete-Time Integrator/1
  Jolt Duration/1 -> Discrete-Time Integrator/2, Data Type Conversion/1
  Jolt Profile/1 -> JoltOutput/1
  Discrete-Time Integrator/1 -> Jolt Profile/1
  Detect Increase/1 -> Jolt Duration/1

== system MotionBaseAdaptersLib/MotionBase/MotionBaseAdapter/MotionBaseProcessing/Dynamic Effects/Acceleration Jolts/Jolt3 ==
  Trigger Jolt : Inport
  Data Type Conversion : DataTypeConversion
  Detect Increase : simulink/Logic and Bit Operations/Detect Increase  vinit=0.0  OutDataTypeStr=boolean
  Discrete-Time Integrator : DiscreteIntegrator  ExternalReset=falling  SampleTime=-1  ICPrevOutput=DiscIntNeverNeededParam  ICPrevScaledInput=DiscIntNeverNeededParam
  Jolt Duration : TimersLib/TimerOffDelay NoInit  UpperSaturationLimit=Duration  SampleTime=-1
      settings: SourceProductName=Sydac Utilities
  Jolt Profile : Lookup_n-D  NumberOfTableDimensions=1  BreakpointsForDimension1=JoltBreakPoints  Table=JoltProfile  ExtrapMethod=Clip  InternalRulePriority=Speed  RndMeth=Simplest  InputSameDT=on
  JoltOutput : Outport
  wires:
  Detect Increase/1 -> Jolt Duration/1
  Discrete-Time Integrator/1 -> Jolt Profile/1
  Jolt Profile/1 -> JoltOutput/1
  Jolt Duration/1 -> Data Type Conversion/1, Discrete-Time Integrator/2
  Data Type Conversion/1 -> Discrete-Time Integrator/1
  Trigger Jolt/1 -> Detect Increase/1

== system MotionBaseAdaptersLib/MotionBase/MotionBaseAdapter/MotionBaseProcessing/ManualAdjustments/ManualPositionAdjustment/DegradedTrackFeel ==
  Linear Velocity : Inport
  RoughnessProfileFactor : Inport  Port=2
  RoughnessProfileSpeedFactor : Inport  Port=3
  RoughnessProfileSpeedSaturation : Inport  Port=4
  RoughnessProfileFrequencyFactor : Inport  Port=5
  Action Port : ActionPort
  AssignZ : Assignment  IndexMode=Zero-based  DiagnosticForDimensions=Warning  IndexOptions=Index vector (dialog)  Indices=2  OutputSizes=1
  Constant : Constant
  DegradedRoughnessGenerator : Subsystem  mask{Variance=0.0001, ClipValue=3, SpeedSaturation=5, Ts=SampleTime}
      mask prompts: SpeedSaturation "Speed Saturation:"; Ts "Simulink:masks:SampleTime_MP"
      mask TypeOptions Ts:
      | Band-Limited
      | White Noise/Ts
      mask DialogControl Ts Prompt: Sample time:
  Selector : Selector  InputPortWidth=3  IndexOptions=Index vector (dialog)  Indices=1  OutputSizes=1
  Zeros : Constant  Value=[0 0 0]
  Out1 : Outport  VectorParamsAs1DForOutWhenUnconnected=off
  wires:
  RoughnessProfileSpeedSaturation/1 -> DegradedRoughnessGenerator/5(SpeedSaturation)
  RoughnessProfileSpeedFactor/1 -> DegradedRoughnessGenerator/4(SpeedFactor)
  Linear Velocity/1 -> Selector/1
  AssignZ/1 -> Out1/1
  DegradedRoughnessGenerator/1(Out1) -> AssignZ/2
  Selector/1 -> DegradedRoughnessGenerator/2(Velocity)  "Forward velocity"
  Zeros/1 -> AssignZ/1
  RoughnessProfileFactor/1 -> DegradedRoughnessGenerator/3(RoughnessAmplitudeFactor)
  Constant/1 -> DegradedRoughnessGenerator/1(Enable)
  RoughnessProfileFrequencyFactor/1 -> DegradedRoughnessGenerator/6(RoughnessProfileFrequencyFactor)

== system MotionBaseAdaptersLib/MotionBase/MotionBaseAdapter/MotionBaseProcessing/ManualAdjustments/ManualPositionAdjustment/EffectSelection ==
  note: Road Effect Override is now just being used to disable road effects if set to a negative value.
      |
      | If we want to try some other profile types we can put in some more options inside the
      | degraded/standard road feel blocks (rather than introduce additional road effects).
  DegradedTrack : Inport
  TrackEffectOverride : Inport  Port=2
  Compare To Zero : simulink/Logic and Bit Operations/Compare To Zero  relop=<  OutDataTypeStr=boolean
  Constant : Constant  Value=TrackEffectType.DegradedTrack
  Constant1 : Constant  Value=TrackEffectType.NoTrackEffect
  Constant2 : Constant  Value=TrackEffectType.StandardTrack
  Switch : Switch  Criteria=u2 > Threshold
  Switch1 : Switch  Criteria=u2 > Threshold
  TrackEffectType : Outport  VectorParamsAs1DForOutWhenUnconnected=off
  wires:
  Constant2/1 -> Switch/3
  Constant/1 -> Switch/1
  Compare To Zero/1 -> Switch1/2
  DegradedTrack/1 -> Switch/2
  Switch1/1 -> TrackEffectType/1
  Constant1/1 -> Switch1/1
  Switch/1 -> Switch1/3
  TrackEffectOverride/1 -> Compare To Zero/1

== system MotionBaseAdaptersLib/MotionBase/MotionBaseAdapter/MotionBaseProcessing/ManualAdjustments/ManualPositionAdjustment/NoTrackFeel ==
  Action Port : ActionPort
  Zeros : Constant  Value=[0 0 0]
  Out1 : Outport  VectorParamsAs1DForOutWhenUnconnected=off
  wires:
  Zeros/1 -> Out1/1

== system MotionBaseAdaptersLib/MotionBase/MotionBaseAdapter/MotionBaseProcessing/ManualAdjustments/ManualPositionAdjustment/StandardTrackFeel ==
  Linear Velocity : Inport
  RoughnessProfileFactor : Inport  Port=2
  RoughnessProfileSpeedFactor : Inport  Port=3
  RoughnessProfileSpeedSaturation : Inport  Port=4
  RoughnessProfileFrequencyFactor : Inport  Port=5
  Action Port : ActionPort
  AssignZ : Assignment  IndexMode=Zero-based  DiagnosticForDimensions=Warning  IndexOptions=Index vector (dialog)  Indices=2  OutputSizes=1
  Constant : Constant
  Selector : Selector  InputPortWidth=3  IndexOptions=Index vector (dialog)  Indices=1  OutputSizes=1
  StandardRoughnessGenerator : Subsystem  mask{Variance=0.0001, ClipValue=3, SpeedSaturation=5, Ts=SampleTime}
      mask prompts: SpeedSaturation "Speed Saturation:"; Ts "Simulink:masks:SampleTime_MP"
      mask TypeOptions Ts:
      | Band-Limited
      | White Noise/Ts
      mask DialogControl Ts Prompt: Sample time:
  Zeros : Constant  Value=[0 0 0]
  Out1 : Outport  VectorParamsAs1DForOutWhenUnconnected=off
  wires:
  RoughnessProfileFrequencyFactor/1 -> StandardRoughnessGenerator/6(RoughnessProfileFrequencyFactor)
  Constant/1 -> StandardRoughnessGenerator/1(Enable)
  RoughnessProfileFactor/1 -> StandardRoughnessGenerator/3(RoughnessAmplitudeFactor)
  Zeros/1 -> AssignZ/1
  Selector/1 -> StandardRoughnessGenerator/2(Velocity)  "Forward velocity"
  StandardRoughnessGenerator/1(Out1) -> AssignZ/2
  AssignZ/1 -> Out1/1
  Linear Velocity/1 -> Selector/1
  RoughnessProfileSpeedFactor/1 -> StandardRoughnessGenerator/4(SpeedFactor)
  RoughnessProfileSpeedSaturation/1 -> StandardRoughnessGenerator/5(SpeedSaturation)

== system MotionBaseAdaptersLib/MotionBase/MotionBaseAdapter/MotionBaseProcessing/ManualAdjustments/ManualPositionAdjustment1/If Action Subsystem ==
  Linear Velocity : Inport
  RoughnessProfileFactor : Inport  Port=2
  RoughnessProfileSpeedFactor : Inport  Port=3
  RoughnessProfileSpeedSaturation : Inport  Port=4
  RoughnessProfileFrequencyFactor : Inport  Port=5
  Action Port : ActionPort
  AssignZ : Assignment  IndexMode=Zero-based  DiagnosticForDimensions=Warning  IndexOptions=Index vector (dialog)  Indices=2  OutputSizes=1
  Constant : Constant
  RoughnessGenerator : Subsystem  mask{Variance=0.0001, ClipValue=3, Ts=SampleTime}
      mask prompts: Ts "Simulink:masks:SampleTime_MP"
      mask TypeOptions Ts:
      | Band-Limited
      | White Noise/Ts
      mask DialogControl Ts Prompt: Sample time:
  Selector : Selector  InputPortWidth=3  IndexOptions=Index vector (dialog)  Indices=1  OutputSizes=1
  Zeros : Constant  Value=[0 0 0]
  Out1 : Outport  VectorParamsAs1DForOutWhenUnconnected=off
  wires:
  RoughnessProfileFactor/1 -> RoughnessGenerator/3(RoughnessAmplitudeFactor)
  Zeros/1 -> AssignZ/1
  Selector/1 -> RoughnessGenerator/2(Velocity)  "Forward velocity"
  RoughnessGenerator/1(Out1) -> AssignZ/2
  AssignZ/1 -> Out1/1
  Linear Velocity/1 -> Selector/1
  RoughnessProfileSpeedFactor/1 -> RoughnessGenerator/4(SpeedFactor)
  RoughnessProfileSpeedSaturation/1 -> RoughnessGenerator/5(SpeedSaturation)
  Constant/1 -> RoughnessGenerator/1(Enable)
  RoughnessProfileFrequencyFactor/1 -> RoughnessGenerator/6(RoughnessProfileFrequencyFactor)

== system MotionBaseAdaptersLib/MotionBase/MotionBaseAdapter/MotionBaseProcessing/ManualAdjustments/ManualPositionAdjustment1/If Action Subsystem1 ==
  Linear Velocity : Inport
  RoughnessProfileFactor : Inport  Port=2
  RoughnessProfileSpeedFactor : Inport  Port=3
  RoughnessProfileSpeedSaturation : Inport  Port=4
  RoughnessProfileFrequencyFactor : Inport  Port=5
  Action Port : ActionPort
  AssignZ : Assignment  IndexMode=Zero-based  DiagnosticForDimensions=Warning  IndexOptions=Index vector (dialog)  Indices=2  OutputSizes=1
  Constant : Constant
  RoughnessGenerator : Subsystem  mask{Variance=0.0001, ClipValue=3, Ts=SampleTime}
      mask prompts: Ts "Simulink:masks:SampleTime_MP"
      mask TypeOptions Ts:
      | Band-Limited
      | White Noise/Ts
      mask DialogControl Ts Prompt: Sample time:
  Selector : Selector  InputPortWidth=3  IndexOptions=Index vector (dialog)  Indices=1  OutputSizes=1
  Zeros : Constant  Value=[0 0 0]
  Out1 : Outport  VectorParamsAs1DForOutWhenUnconnected=off
  wires:
  RoughnessProfileSpeedSaturation/1 -> RoughnessGenerator/5(SpeedSaturation)
  RoughnessProfileSpeedFactor/1 -> RoughnessGenerator/4(SpeedFactor)
  Linear Velocity/1 -> Selector/1
  AssignZ/1 -> Out1/1
  RoughnessGenerator/1(Out1) -> AssignZ/2
  Selector/1 -> RoughnessGenerator/2(Velocity)  "Forward velocity"
  Zeros/1 -> AssignZ/1
  RoughnessProfileFactor/1 -> RoughnessGenerator/3(RoughnessAmplitudeFactor)
  Constant/1 -> RoughnessGenerator/1(Enable)
  RoughnessProfileFrequencyFactor/1 -> RoughnessGenerator/6(RoughnessProfileFrequencyFactor)

== system MotionBaseAdaptersLib/MotionBase/MotionBaseAdapter/MotionBaseProcessing/ManualAdjustments/ManualPositionAdjustment1/If Action Subsystem2 ==
  Action Port : ActionPort
  Zeros : Constant  Value=[0 0 0]
  Out1 : Outport  VectorParamsAs1DForOutWhenUnconnected=off
  wires:
  Zeros/1 -> Out1/1
